simulink model "nonlinearlqg"  (R2018b)
settings: Solver=VariableStepAuto  StartTime=0.0  StopTime=100  RelTol=1e-3
values from neighbouring files (symbols this model uses):
  Ac = A-L1*C1    [mycode.m]
  Bc = [B L1]    [mycode.m]
  C1 = [1 0 0 0 0 0]    [mycode.m]
  Cc = eye(6)    [mycode.m]
  Dc = 0*[B L1]    [mycode.m]
undefined symbols (not defined in the file or in its folder): K
settings Model: Creator=abhin  LastModifiedBy=abhin
settings DebuggingCC: UnderSpecifiedDimensionMsg=warning

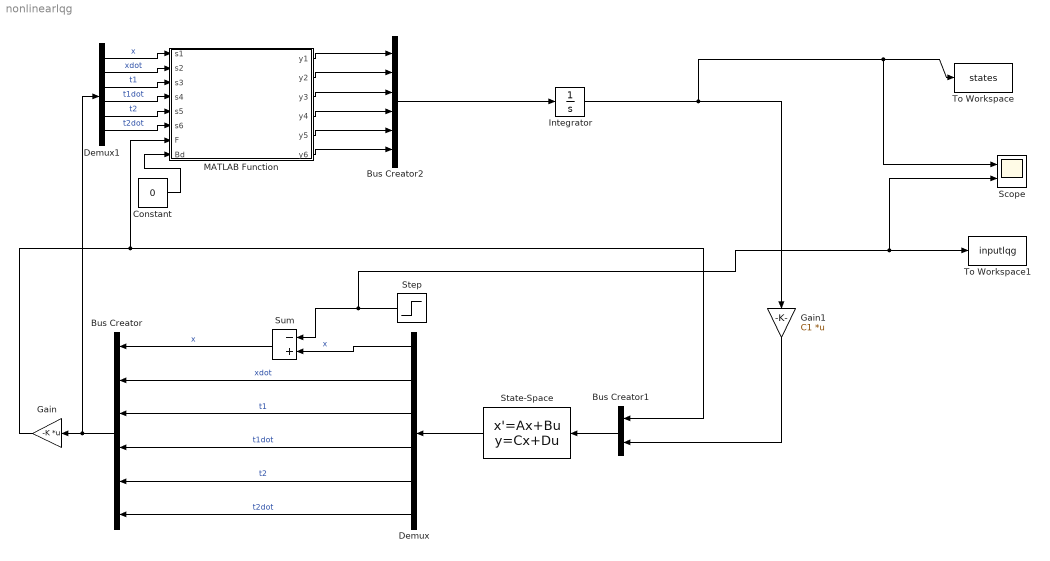
== system nonlinearlqg ==
  Bus Creator : BusCreator  Inputs=6
  Bus Creator1 : BusCreator  Inputs=2
  Bus Creator2 : BusCreator  Inputs=6
  Constant : Constant  Value=0
  Demux : Demux  Outputs=6
  Demux1 : Demux  Outputs=6
  Gain : Gain  Gain=-K  Multiplication=Matrix(K*u)
  Gain1 : Gain  Gain=C1  Multiplication=Matrix(K*u)
  Integrator : Integrator  InitialCondition=[0;0;0;0;0;0]
  MATLAB Function : MATLAB Function  TreatAsAtomicUnit=on
  Scope : Scope  NumInputPorts=2
  State-Space : StateSpace  A=Ac  B=Bc  C=Cc  D=Dc  InitialCondition=0
  Step : Step  Time=20  SampleTime=0
  Sum : Sum  Inputs=-+
  To Workspace : ToWorkspace  VariableName=states  SampleTime=-1
  To Workspace1 : ToWorkspace  VariableName=inputlqg  SampleTime=-1
  wires:
  State-Space/1 -> Demux/1
  Sum/1 -> Bus Creator/1  "x"
  Demux/2 -> Bus Creator/2  "xdot"
  Demux/3 -> Bus Creator/3  "t1"
  Demux/4 -> Bus Creator/4  "t1dot"
  Demux/5 -> Bus Creator/5  "t2"
  Demux/6 -> Bus Creator/6  "t2dot"
  Step/1 -> Scope/2, To Workspace1/1, Sum/1
  Demux/1 -> Sum/2  "x"
  Bus Creator/1 -> Demux1/1, Gain/1
  Gain/1 -> MATLAB Function/7(F), Bus Creator1/1
  Gain1/1 -> Bus Creator1/2
  Bus Creator1/1 -> State-Space/1
  Integrator/1 -> Scope/1, To Workspace/1, Gain1/1
  MATLAB Function/1(y1) -> Bus Creator2/1
  MATLAB Function/2(y2) -> Bus Creator2/2
  MATLAB Function/3(y3) -> Bus Creator2/3
  MATLAB Function/4(y4) -> Bus Creator2/4
  MATLAB Function/5(y5) -> Bus Creator2/5
  MATLAB Function/6(y6) -> Bus Creator2/6
  Bus Creator2/1 -> Integrator/1
  Demux1/1 -> MATLAB Function/1(s1)  "x"
  Demux1/2 -> MATLAB Function/2(s2)  "xdot"
  Demux1/3 -> MATLAB Function/3(s3)  "t1"
  Demux1/4 -> MATLAB Function/4(s4)  "t1dot"
  Demux1/5 -> MATLAB Function/5(s5)  "t2"
  Demux1/6 -> MATLAB Function/6(s6)  "t2dot"
  Constant/1 -> MATLAB Function/8(Bd)

== matlab function nonlinearlqg/MATLAB Function ==
  data: s1 input; y1 output; s2 input; s3 input; s4 input; s5 input; s6 input; F input; y2 output; y3 output; y4 output; y5 output; y6 output; Bd input
function [y1,y2,y3,y4,y5,y6]  = nonlinearlqg(s1,s2,s3,s4,s5,s6,F,Bd)

params.M = 1000; %mass of cart 1000
params.m1 = 100; %mass of bob 1 100
params.m2 = 100; %mass of bob 2 100
params.l1 = 20;  %length of link of first pendulum 20
params.l2 = 10;  %length of link of second pendulum 10
params.g = 10; %acceleration due to gravitaion 9.81

x = s1;
x_dot = s2;
t1 = s3;
t1_dot = s4;
t2 = s5;
t2_dot = s6;
uD = 1;

s_dot = zeros(6,1);
s_dot1 = x_dot + Bd*uD;
s_dot2 = (F - params.m1*params.g*sin(2*t1)/2 - params.m2*params.g*sin(2*t2)/2 - params.m1*params.l1*sin(t1)*(t1_dot)^2 - params.m2*params.l2*sin(t2)*(t2_dot)^2)/(params.M + params.m1*(sin(t1)^2) + params.m2*(sin(t2)^2))+Bd*uD;
s_dot3 = t1_dot+Bd*uD;
s_dot4 = (1/params.l1)*(cos(t1)*(F - params.m1*params.g*sin(2*t1)/2 - params.m2*params.g*sin(2*t2)/2 - params.m1*params.l1*sin(t1)*(t1_dot)^2 - params.m2*params.l2*sin(t2)*(t2_dot)^2)/(params.M + params.m1*(sin(t1)^2) + params.m2*(sin(t2)^2)) - params.g*sin(t1))+Bd*uD;
s_dot5 = t2_dot+Bd*uD;
s_dot6 = (1/params.l2)*(cos(t2)*(F - params.m1*params.g*sin(2*t1)/2 - params.m2*params.g*sin(2*t2)/2  - params.m1*params.l1*sin(t1)*(t1_dot)^2 - params.m2*params.l2*sin(t2)*(t2_dot)^2)/(params.M + params.m1*(sin(t1)^2) + params.m2*(sin(t2)^2)) - params.g*sin(t2))+Bd*uD;

y1 = s_dot1;
y2 = s_dot2;
y3 = s_dot3;
y4 = s_dot4;
y5 = s_dot5;
y6 = s_dot6;
